simulink model "DC_Oserver"  (R2015a)
settings: Solver=ode45  StartTime=0.0  StopTime=0.1  MaxStep=0.0000001  MinStep=0.00000001  RelTol=1e-3
libraries: powerlib x9, simulink_extras x7, simulink x3
settings Model: Creator=hp  LastModifiedBy=hp
settings SolverCC: ZeroCrossControl=DisableAll

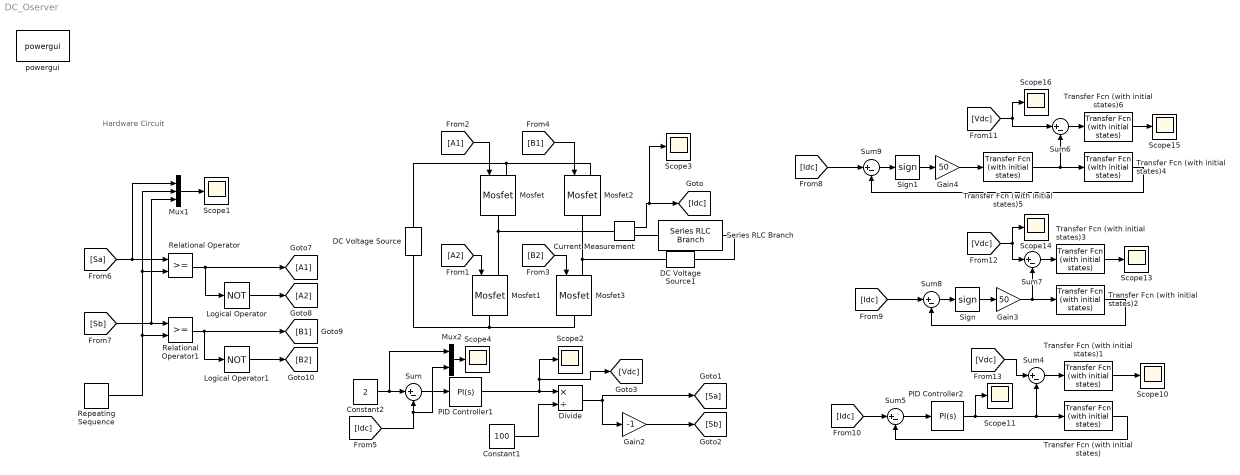
== system DC_Oserver ==
  note: Hardware Circuit
  Constant1 : Constant  Value=100
  Constant2 : Constant  Value=2
  Current Measurement : powerlib/Measurements/Current Measurement  PhasorSimulation=off  OutputType=Complex  PSBequivalent=0
  DC Voltage Source : powerlib/Electrical Sources/DC Voltage Source  Amplitude=100  Measurements=None
  DC Voltage Source1 : powerlib/Electrical Sources/DC Voltage Source  Amplitude=1  Measurements=None
  Divide : Product  Inputs=*/
  Gain2 : Gain  Gain=-1
  Gain3 : Gain  Gain=50
  Gain4 : Gain  Gain=50
  Logical Operator : Logic  Operator=NOT  Inputs=1  AllPortsSameDT=off  OutDataTypeStr=boolean
  Logical Operator1 : Logic  Operator=NOT  Inputs=1  AllPortsSameDT=off  OutDataTypeStr=boolean
  Mosfet{,1..3} (4 alike) : powerlib/Power Electronics/Mosfet  Ron=0.0001  Lon=0  Rd=0.0001  Vfd=0  IC=0  Rs=1e5  Cs=inf  Measurements=off
  Mux1 : Mux  Inputs=3
  Mux2 : Mux  Inputs=2
  PID Controller1 : simulink/Continuous/PID Controller  Controller=PI  TimeDomain=Continuous-time  SampleTime=-1  IntegratorMethod=Forward Euler  FilterMethod=Forward Euler  Form=Parallel  UseFilter=on  ControllerParametersSource=internal  P=40  I=15000  D=0  N=100  InitialConditionSource=internal  InitialConditionForIntegrator=0  InitialConditionForFilter=0  ExternalReset=none  LimitOutput=on  UpperSaturationLimit=100  LowerSaturationLimit=-100  LinearizeAsGain=on  AntiWindupMode=none  Kb=1  TrackingMode=off  Kt=1  PParamMin=[]  PParamMax=[]  IParamMin=[]  IParamMax=[]  DParamMin=[]  DParamMax=[]  NParamMin=[]  NParamMax=[]  KbParamMin=[]  KbParamMax=[]  KtParamMin=[]  KtParamMax=[]  POutMin=[]  POutMax=[]  IOutMin=[]  IOutMax=[]  DOutMin=[]  DOutMax=[]  NOutMin=[]  NOutMax=[]  KbOutMin=[]  KbOutMax=[]  KtOutMin=[]  KtOutMax=[]  IntegratorOutMin=[]  IntegratorOutMax=[]  FilterOutMin=[]  FilterOutMax=[]  SumOutMin=[]  SumOutMax=[]  SumI1OutMin=[]  SumI1OutMax=[]  SumI2OutMin=[]  SumI2OutMax=[]  SumI3OutMin=[]  SumI3OutMax=[]  SumDOutMin=[]  SumDOutMax=[]  SaturationOutMin=[]  SaturationOutMax=[]  IntegratorContinuousStateAttributes=''  IntegratorStateMustResolveToSignalObject=off  IntegratorRTWStateStorageClass=Auto  FilterContinuousStateAttributes=''  FilterStateMustResolveToSignalObject=off  FilterRTWStateStorageClass=Auto  DifferentiatorICPrevScaledInput=0  DifferentiatorOutMin=[]  DifferentiatorOutMax=[]
  PID Controller2 : simulink/Continuous/PID Controller  Controller=PI  TimeDomain=Continuous-time  SampleTime=-1  IntegratorMethod=Forward Euler  FilterMethod=Forward Euler  Form=Parallel  UseFilter=on  ControllerParametersSource=internal  P=40  I=15000  D=0  N=100  InitialConditionSource=internal  InitialConditionForIntegrator=0  InitialConditionForFilter=0  ExternalReset=none  LimitOutput=on  UpperSaturationLimit=100  LowerSaturationLimit=-100  LinearizeAsGain=on  AntiWindupMode=none  Kb=1  TrackingMode=off  Kt=1  PParamMin=[]  PParamMax=[]  IParamMin=[]  IParamMax=[]  DParamMin=[]  DParamMax=[]  NParamMin=[]  NParamMax=[]  KbParamMin=[]  KbParamMax=[]  KtParamMin=[]  KtParamMax=[]  POutMin=[]  POutMax=[]  IOutMin=[]  IOutMax=[]  DOutMin=[]  DOutMax=[]  NOutMin=[]  NOutMax=[]  KbOutMin=[]  KbOutMax=[]  KtOutMin=[]  KtOutMax=[]  IntegratorOutMin=[]  IntegratorOutMax=[]  FilterOutMin=[]  FilterOutMax=[]  SumOutMin=[]  SumOutMax=[]  SumI1OutMin=[]  SumI1OutMax=[]  SumI2OutMin=[]  SumI2OutMax=[]  SumI3OutMin=[]  SumI3OutMax=[]  SumDOutMin=[]  SumDOutMax=[]  SaturationOutMin=[]  SaturationOutMax=[]  IntegratorContinuousStateAttributes=''  IntegratorStateMustResolveToSignalObject=off  IntegratorRTWStateStorageClass=Auto  FilterContinuousStateAttributes=''  FilterStateMustResolveToSignalObject=off  FilterRTWStateStorageClass=Auto  DifferentiatorICPrevScaledInput=0  DifferentiatorOutMin=[]  DifferentiatorOutMax=[]
  Relational Operator : RelationalOperator  OutDataTypeStr=boolean
  Relational Operator1 : RelationalOperator  OutDataTypeStr=boolean
  Repeating Sequence : simulink/Sources/Repeating Sequence  rep_seq_t=[0 0.25 0.5 0.75 1]/20000  rep_seq_y=[0 1 0 -1 0]
  Scope{1..4,10..11,13..16} (10 alike) : Scope
      Scope1 settings: TimeRange=0.1  YMin=-1  YMax=1
      Scope10 settings: YMin=0.1675  YMax=0.2  SaveName=ScopeData9
      Scope11 settings: YMin=-0.5  SaveName=ScopeData10
      Scope13 settings: YMin=0.165  YMax=0.2  SaveName=ScopeData12
      Scope14 settings: YMin=-0.5  SaveName=ScopeData13
      Scope15 settings: YMin=-0.1  YMax=2  SaveName=ScopeData14
      Scope16 settings: YMin=-0.5  SaveName=ScopeData15
      Scope2 settings: TimeRange=0.1  YMin=3.85  YMax=4.8
      Scope3 settings: TimeRange=0.1  YMin=1.91  YMax=1.9525  SaveName=ScopeData2
      Scope4 settings: TimeRange=0.1  YMin=2.96  YMax=3.04  SaveName=ScopeData3
  Series RLC Branch : powerlib/Elements/Series RLC Branch  LConnTagsString=__new0  RConnTagsString=__new0  BranchType=RL  Resistance=2.07  Inductance=5e-3  SetiL0=off  InitialCurrent=0  Capacitance=1e-6  Setx0=off  InitialVoltage=0  Measurements=None
  Sign : Signum
  Sign1 : Signum
  Sum{,4..9} (7 alike) : Sum  Inputs=|+-
  Transfer Fcn (with initial states) : simulink_extras/Additional Linear/Transfer Fcn (with initial states)  N=[1]  D=[0.005 2.07]  X0=0
  Transfer Fcn (with initial states)1 : simulink_extras/Additional Linear/Transfer Fcn (with initial states)  N=[2*3.14*500]  D="[1  2*3.14*500]"  X0=0
  Transfer Fcn (with initial states)2 : simulink_extras/Additional Linear/Transfer Fcn (with initial states)  N=[1]  D=[0.005 2.07]  X0=0
  Transfer Fcn (with initial states)3 : simulink_extras/Additional Linear/Transfer Fcn (with initial states)  N=[2*3.14*50]  D="[1  2*3.14*50]"  X0=0
  Transfer Fcn (with initial states)4 : simulink_extras/Additional Linear/Transfer Fcn (with initial states)  N=[1]  D=[0.005 2.07]  X0=0
  Transfer Fcn (with initial states)5 : simulink_extras/Additional Linear/Transfer Fcn (with initial states)  N=[2*3.14*5000]  D="[1  2*3.14*5000]"  X0=0
  Transfer Fcn (with initial states)6 : simulink_extras/Additional Linear/Transfer Fcn (with initial states)  N=[2*3.14*50]  D="[1  2*3.14*50]"  X0=0
  powergui : powerlib/powergui  Priority=1  SimulationMode=Discrete  SolverType=Tustin/Backward Euler (TBE)  SampleTime=1e-7  frequency=60  SPID=off  DisableSnubberDevices=off  DisableRonSwitches=off  DisableVfSwitches=off  SwTol=0  DisplayEquations=off  Interpol=off  methode=off  Ts=100  FunctionMessages=off  echomessages=off  HookPort=off  EnableUseOfTLC=off  x0status=blocks  frequencyindice=0  Pbase=100e6  ErrMax=1e-4  Iterations=50  UnitsV=kV  UnitsW=MW  buscounter=0  RestoreLinks=warning  ResistiveCurrentMeasurement=off  Frange=[0:2:500]  Ylog=off  Xlog=on  ShowGrid=off  save=off  variable=ZData  structure=0  ZoomFFT=off  StartTime=0.0  cycles=1  DisplayStyle=1  fundamental=60  FreqAxis=off  MaxFrequency=1000  frequencyindicesteady=1  RmsSteady=1  display=off
  wires:
  [B1] -> Mosfet2/1
  [B2] -> Mosfet3/1
  [A2] -> Mosfet1/1
  [A1] -> Mosfet/1
  [Sb] -> Mux1/3, Relational Operator1/1
  Relational Operator/1 -> Logical Operator/1, [A1]
  Logical Operator/1 -> [A2]
  Relational Operator1/1 -> Logical Operator1/1, [B1]
  Logical Operator1/1 -> [B2]
  Divide/1 -> Gain2/1, [Sa]
  Constant1/1 -> Divide/2
  Gain2/1 -> [Sb]
  [Sa] -> Mux1/1, Relational Operator/1
  Repeating Sequence/1 -> Relational Operator1/2, Mux1/2, Relational Operator/2
  Mux1/1 -> Scope1/1
  PID Controller1/1 -> Scope2/1, [Vdc], Divide/1
  Current Measurement/1 -> Scope3/1, [Idc]
  Sum/1 -> PID Controller1/1
  Mux2/1 -> Scope4/1
  [Idc] -> Mux2/2, Sum/2
  Constant2/1 -> Mux2/1, Sum/1
  Sum9/1 -> Sign1/1
  [Idc] -> Sum9/1
  Transfer Fcn (with initial states)4/1 -> Sum9/2
  Transfer Fcn (with initial states)6/1 -> Scope15/1
  Sum6/1 -> Transfer Fcn (with initial states)6/1
  [Vdc] -> Scope16/1, Sum6/1
  Sign1/1 -> Gain4/1
  Gain4/1 -> Transfer Fcn (with initial states)5/1
  Transfer Fcn (with initial states)5/1 -> Sum6/2, Transfer Fcn (with initial states)4/1
  Sum5/1 -> PID Controller2/1
  PID Controller2/1 -> Transfer Fcn (with initial states)/1, Sum4/2, Scope11/1
  [Idc] -> Sum5/1
  Transfer Fcn (with initial states)/1 -> Sum5/2
  Transfer Fcn (with initial states)1/1 -> Scope10/1
  Sum4/1 -> Transfer Fcn (with initial states)1/1
  [Vdc] -> Sum4/1
  Sum8/1 -> Sign/1
  [Idc] -> Sum8/1
  Transfer Fcn (with initial states)2/1 -> Sum8/2
  Transfer Fcn (with initial states)3/1 -> Scope13/1
  Sum7/1 -> Transfer Fcn (with initial states)3/1
  [Vdc] -> Scope14/1, Sum7/1
  Sign/1 -> Gain3/1
  Gain3/1 -> Transfer Fcn (with initial states)2/1, Sum7/2
  connections:
  Mosfet/RConn1 -- Current Measurement/LConn1 -- Mosfet1/LConn1
  Mosfet3/LConn1 -- DC Voltage Source1/LConn1 -- Mosfet2/RConn1
  Mosfet3/RConn1 -- DC Voltage Source/LConn1 -- Mosfet1/RConn1
  Mosfet/LConn1 -- DC Voltage Source/RConn1 -- Mosfet2/LConn1
  Current Measurement/RConn1 -- Series RLC Branch/LConn1
  DC Voltage Source1/RConn1 -- Series RLC Branch/RConn1
